simulink model "manual_steer"  (R2022b)
settings: Solver=ode4  StartTime=0.0  StopTime=100  RelTol=1e-3
model workspace (MAT data in the model file):
  x2xx = 0
undefined symbols (not defined in the file or in its folder): axle_rate_limit, BRAKE, brake_lag, brake_rate, DRIVE, KDspd, KIspd, KPspd, Lspd, Nspd, PARSa, PARSu, Q0, QD0, RW, Tb, Tmc, TOTALMASS, Tst, Uspd, v_ref
libraries: CarMaker4SL x72, slpidlib x4, TruckMaker4SL x1, simulink x1
(part 1 of 5)
settings Model: Creator=DJW  LastModifiedBy=14668
settings DebuggingCC: UnconnectedInputMsg=warning  UnconnectedOutputMsg=warning  UnconnectedLineMsg=warning  SFMachineParentedDataDiag=warning
settings ModelReferenceCC: EnableRefExpFcnMdlSchedulingChecks=on

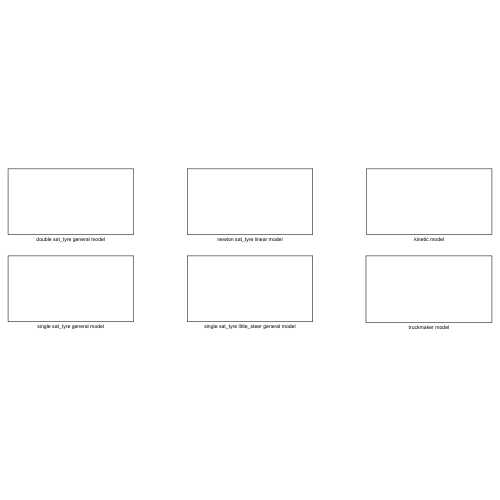
[thumbnail: Simulink's stored preview of the top-level diagram]
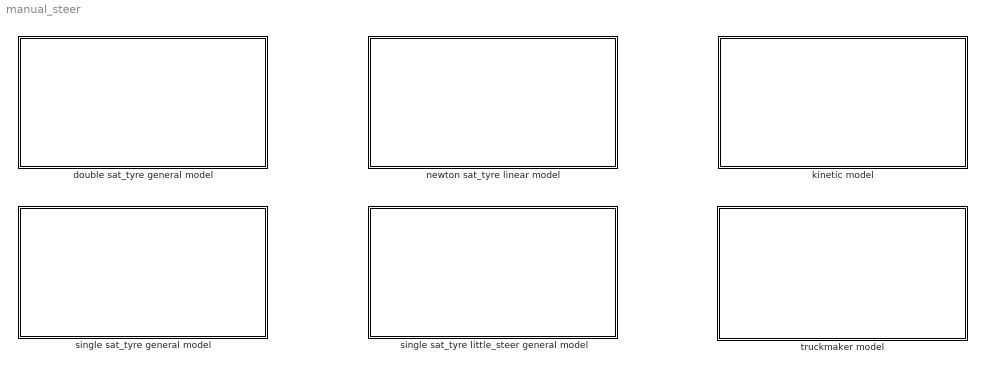
== system manual_steer ==
  double sat_tyre general model : Subsystem
  kinetic model : Subsystem
  newton sat_tyre linear model : Subsystem
  single sat_tyre general model : Subsystem
  single sat_tyre little_steer general model : Subsystem
  truckmaker model : Subsystem

== system manual_steer/double sat_tyre general model ==
  " Motion Controller" : Subsystem  SystemSampleTime=Tmc
  " Motion Controller1" : Subsystem  Commented=on  SystemSampleTime=Tmc
  Clock : Clock
  To Workspace2 : ToWorkspace  VariableName=time  SampleTime=-1
  To Workspace4 : ToWorkspace  VariableName=steer_out  SampleTime=-1
  double-general-lineartyre-nonlinear-constant-matrix : Subsystem  Commented=on
  double-general-lineartyre-variable : Subsystem
  double-general-nonlineartyre-nonlinear-constant-matrix : Subsystem  Commented=on
  double-general-nonlineartyre-nonlinear-variable-matrix : Subsystem  Commented=on
  proc : Subsystem
  single-general-lineartyre-nonlinear-variable-matrix : Subsystem  Commented=on
  wires:
  Clock/1 -> To Workspace2/1
  " Motion Controller"/1(steer6) -> To Workspace4/1, double-general-lineartyre-variable/1(steer)
  " Motion Controller"/2(Fx) -> double-general-lineartyre-variable/2(Fx_in)

== system manual_steer/kinetic model ==
  " Motion Controller No Fx" : Subsystem  SystemSampleTime=Tmc
  Clock : Clock
  To Workspace2 : ToWorkspace  VariableName=time_kinetic  SampleTime=-1
  To Workspace4 : ToWorkspace  VariableName=steer_out_kinetic  SampleTime=-1
  kinetic linear : Subsystem
  proc : Subsystem
  wires:
  Clock/1 -> To Workspace2/1
  " Motion Controller No Fx"/1(steer) -> To Workspace4/1, kinetic linear/1(steer)

== system manual_steer/newton sat_tyre linear model ==
  " Motion Controller No Fx" : Subsystem  SystemSampleTime=Tmc
  Clock : Clock
  To Workspace2 : ToWorkspace  VariableName=time_newton  SampleTime=-1
  To Workspace4 : ToWorkspace  VariableName=steer_out_newton  SampleTime=-1
  newton sat_tyre linear : Subsystem
  proc : Subsystem
  wires:
  Clock/1 -> To Workspace2/1
  " Motion Controller No Fx"/1(steer) -> To Workspace4/1, newton sat_tyre linear/1(steer)

== system manual_steer/single sat_tyre general model ==
  " Motion Controller" : Subsystem  SystemSampleTime=Tmc
  Clock : Clock
  To Workspace2 : ToWorkspace  VariableName=time_single  SampleTime=-1
  To Workspace4 : ToWorkspace  VariableName=steer_out_single  SampleTime=-1
  proc : Subsystem
  single-general-lineartyre-variable : Subsystem
  wires:
  Clock/1 -> To Workspace2/1
  " Motion Controller"/1(steer6) -> To Workspace4/1, single-general-lineartyre-variable/1(steer)
  " Motion Controller"/2(Fx) -> single-general-lineartyre-variable/2(Fx_in)

== system manual_steer/single sat_tyre little_steer general model ==
  " Motion Controller" : Subsystem  SystemSampleTime=Tmc
  Clock : Clock
  To Workspace2 : ToWorkspace  VariableName=time_single_littles  SampleTime=-1
  To Workspace4 : ToWorkspace  VariableName=steer_out_single_littles  SampleTime=-1
  proc : Subsystem
  single-general-lineartyre-little steer-variable : Subsystem
  wires:
  Clock/1 -> To Workspace2/1
  " Motion Controller"/1(steer6) -> To Workspace4/1, single-general-lineartyre-little steer-variable/1(steer)
  " Motion Controller"/2(Fx) -> single-general-lineartyre-little steer-variable/2(Fx_in)

== system manual_steer/truckmaker model ==
  Edit Model Configuration : TruckMaker4SL/Edit Model Configuration  SFunctionModules=''
  Open TruckMaker GUI : Subsystem  LoadFcn=if ~length(which('cmself')), cmenv; end
      settings: OpenFcn=cmblockmagic('gui_fix_display'); TM_Simulink
      mask Display: image(imread('TruckMakerGUI.png'));
  TruckMaker : Subsystem  TreatAsAtomicUnit=on
      mask Display: image(imread('TruckMakerSys.png'));

== system manual_steer/double sat_tyre general model/ Motion Controller ==
  Rate Transition{3..6} (4 alike) : RateTransition
  discrete-time subsystem : Subsystem  TreatAsAtomicUnit=on  SystemSampleTime=Tmc
  steer6 : Outport
  Fx : Outport  Port=2
  wires:
  [q_] -> Rate Transition4/1
  Rate Transition5/1 -> Fx/1
  Rate Transition6/1 -> steer6/1
  [qd_] -> Rate Transition3/1
  discrete-time subsystem/1(steer) -> Rate Transition6/1
  Rate Transition4/1 -> discrete-time subsystem/1(q_in)
  Rate Transition3/1 -> discrete-time subsystem/2(qd_in)
  discrete-time subsystem/2(Fx_input) -> Rate Transition5/1

== system manual_steer/double sat_tyre general model/ Motion Controller1 ==
  Rate Transition6 : RateTransition
  discrete-time subsystem : Subsystem  TreatAsAtomicUnit=on  SystemSampleTime=Tmc
  steer6 : Outport
  wires:
  Rate Transition6/1 -> steer6/1
  discrete-time subsystem/1(steer) -> Rate Transition6/1

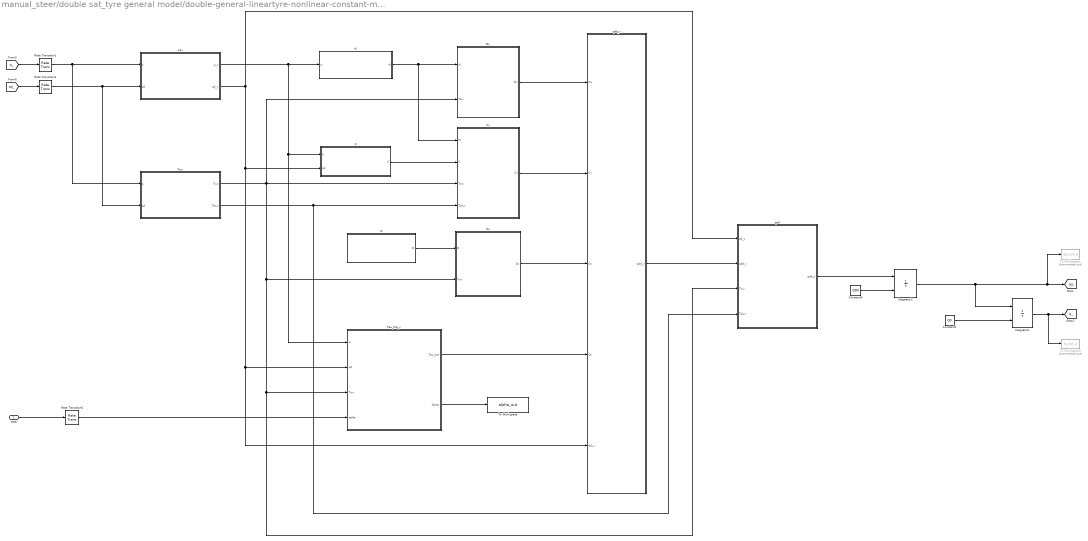
== system manual_steer/double sat_tyre general model/double-general-lineartyre-nonlinear-constant-matrix ==
  steer : Inport
  C : MATLAB Function  TreatAsAtomicUnit=on
  Constant1 : Constant  Value=Q0
  Constant4 : Constant  Value=QD0
  Cv : MATLAB Function  TreatAsAtomicUnit=on
  D : MATLAB Function  TreatAsAtomicUnit=on
  Dv : MATLAB Function  TreatAsAtomicUnit=on
  Integrator1 : Integrator  InitialConditionSource=external  InitialCondition=Q0
  Integrator2 : Integrator  InitialConditionSource=external  InitialCondition=zeros(5,1)
  M : MATLAB Function  TreatAsAtomicUnit=on
  Mv : MATLAB Function  TreatAsAtomicUnit=on
  Rate Transition1 : RateTransition
  Rate Transition2 : RateTransition
  Rate Transition6 : RateTransition
  Tau_tire_v : MATLAB Function  TreatAsAtomicUnit=on
  To Workspace : ToWorkspace  VariableName=alpha_out  SampleTime=-1
  To Workspace1 : ToWorkspace  Commented=on  VariableName=qd_out_4  SampleTime=-1
  To Workspace3 : ToWorkspace  Commented=on  VariableName=q_out_4  SampleTime=-1
  Twv : MATLAB Function  TreatAsAtomicUnit=on
  qdd : MATLAB Function  TreatAsAtomicUnit=on
  qdd_v : MATLAB Function  TreatAsAtomicUnit=on
  w2v : MATLAB Function  TreatAsAtomicUnit=on
  tag scope: q_=global, qd_=global
  wires:
  M/1(M) -> Cv/1(M), Mv/1(M)
  [q_] -> Rate Transition1/1
  [qd_] -> Rate Transition2/1
  Twv/1(Twv) -> qdd/3(Twv), Tau_tire_v/3(Twv), Dv/2(Twv), Cv/3(Twv), Mv/2(Twv)
  C/1(C) -> Cv/2(C)
  Twv/2(Tdwv) -> qdd/4(Tdwv), Cv/4(Tdwv)
  D/1(D) -> Dv/1(D)
  steer/1 -> Rate Transition6/1
  w2v/1(q_v) -> M/1(q), Tau_tire_v/1(q), C/1(q)
  Mv/1(Mv) -> qdd_v/1(Mv)
  Dv/1(Dv) -> qdd_v/3(Dv)
  Cv/1(Cv) -> qdd_v/2(Cv)
  Tau_tire_v/1(Tau_tire) -> qdd_v/4(Qv)
  w2v/2(qd_v) -> qdd/1(qd_v), Tau_tire_v/2(qd), qdd_v/5(qd_v), C/2(qd)
  qdd_v/1(qdd_v) -> qdd/2(qdd_v)
  qdd/1(qdd_n) -> Integrator2/1
  Integrator1/1 -> To Workspace3/1, [q_]
  Integrator2/1 -> To Workspace1/1, [qd_], Integrator1/1
  Tau_tire_v/2(Alpha) -> To Workspace/1
  Constant4/1 -> Integrator2/2
  Constant1/1 -> Integrator1/2
  Rate Transition6/1 -> Tau_tire_v/4(delta)
  Rate Transition1/1 -> Twv/1(q), w2v/1(q)
  Rate Transition2/1 -> Twv/2(qd), w2v/2(qd)

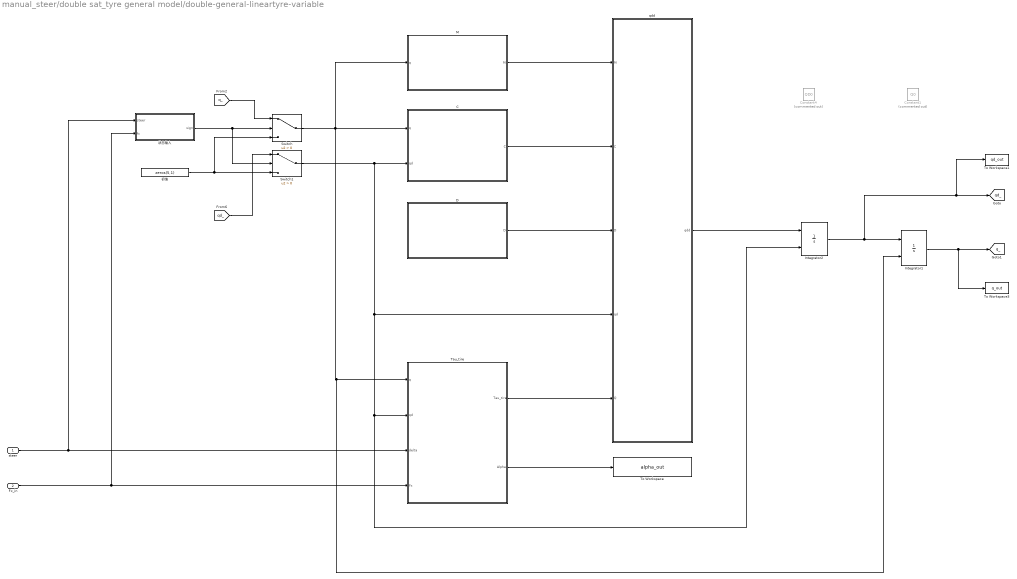
== system manual_steer/double sat_tyre general model/double-general-lineartyre-variable ==
  steer : Inport
  Fx_in : Inport  Port=2
  C : MATLAB Function  TreatAsAtomicUnit=on
  Constant1 : Constant  Commented=on  Value=Q0
  Constant4 : Constant  Commented=on  Value=QD0
  D : MATLAB Function  TreatAsAtomicUnit=on
  Integrator1 : Integrator  InitialConditionSource=external  InitialCondition=Q0
  Integrator2 : Integrator  InitialConditionSource=external  InitialCondition=zeros(5,1)
  M : MATLAB Function  TreatAsAtomicUnit=on
  Switch : Switch  Criteria=u2 > Threshold  SaturateOnIntegerOverflow=off  InputSameDT=off
  Switch1 : Switch  Criteria=u2 > Threshold  SaturateOnIntegerOverflow=off  InputSameDT=off
  Tau_tire : MATLAB Function  TreatAsAtomicUnit=on
  To Workspace : ToWorkspace  VariableName=alpha_out  SampleTime=-1
  To Workspace1 : ToWorkspace  VariableName=qd_out  SampleTime=-1
  To Workspace3 : ToWorkspace  VariableName=q_out  SampleTime=-1
  qdd : MATLAB Function  TreatAsAtomicUnit=on
  初值 : Constant  Value=zeros(5,1)
  状态输入 : MATLAB Function  TreatAsAtomicUnit=on
  tag scope: q_=global, qd_=global
  wires:
  Integrator1/1 -> To Workspace3/1, [q_]
  Fx_in/1 -> 状态输入/2(fx), Tau_tire/4(Fx)
  steer/1 -> 状态输入/1(steer), Tau_tire/3(delta)
  Tau_tire/2(Alpha) -> To Workspace/1
  qdd/1(qdd) -> Integrator2/1
  Integrator2/1 -> To Workspace1/1, [qd_], Integrator1/1
  M/1(M) -> qdd/1(M)
  C/1(C) -> qdd/2(C)
  Tau_tire/1(Tau_tire) -> qdd/5(Q)
  D/1(D) -> qdd/3(D)
  状态输入/1(sign) -> Switch1/2, Switch/2
  初值/1 -> Switch/3, Switch1/3
  Switch/1 -> Integrator1/2, Tau_tire/1(q), M/1(q), C/1(q)
  Switch1/1 -> Integrator2/2, Tau_tire/2(qd), qdd/4(qd), C/2(qd)
  [qd_] -> Switch1/1
  [q_] -> Switch/1

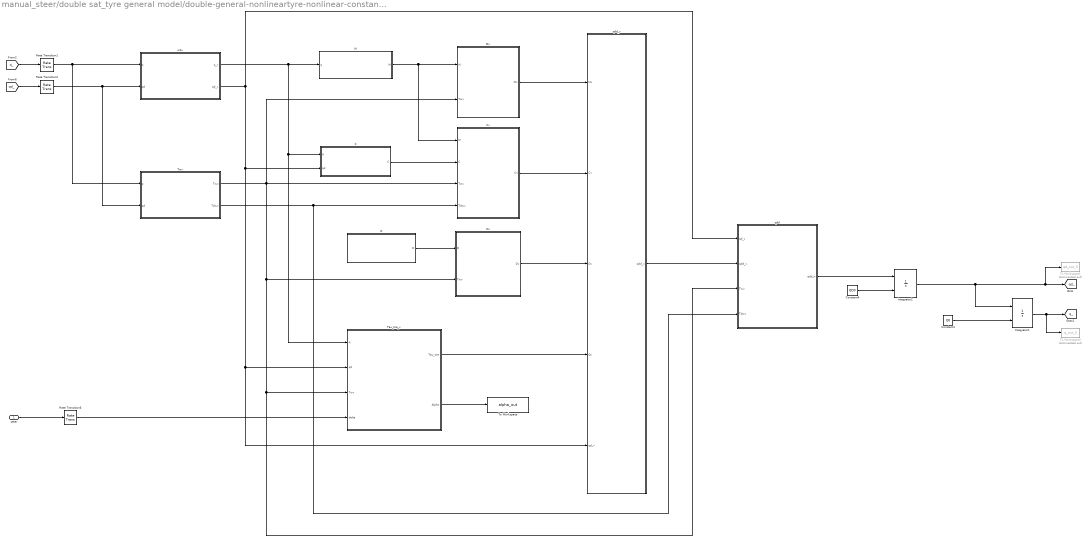
== system manual_steer/double sat_tyre general model/double-general-nonlineartyre-nonlinear-constant-matrix ==
  steer : Inport
  C : MATLAB Function  TreatAsAtomicUnit=on
  Constant1 : Constant  Value=Q0
  Constant4 : Constant  Value=QD0
  Cv : MATLAB Function  TreatAsAtomicUnit=on
  D : MATLAB Function  TreatAsAtomicUnit=on
  Dv : MATLAB Function  TreatAsAtomicUnit=on
  Integrator1 : Integrator  InitialConditionSource=external  InitialCondition=Q0
  Integrator2 : Integrator  InitialConditionSource=external  InitialCondition=zeros(5,1)
  M : MATLAB Function  TreatAsAtomicUnit=on
  Mv : MATLAB Function  TreatAsAtomicUnit=on
  Rate Transition1 : RateTransition
  Rate Transition2 : RateTransition
  Rate Transition6 : RateTransition
  Tau_tire_v : MATLAB Function  TreatAsAtomicUnit=on
  To Workspace : ToWorkspace  VariableName=alpha_out  SampleTime=-1
  To Workspace1 : ToWorkspace  Commented=on  VariableName=qd_out_5  SampleTime=-1
  To Workspace3 : ToWorkspace  Commented=on  VariableName=q_out_5  SampleTime=-1
  Twv : MATLAB Function  TreatAsAtomicUnit=on
  qdd : MATLAB Function  TreatAsAtomicUnit=on
  qdd_v : MATLAB Function  TreatAsAtomicUnit=on
  w2v : MATLAB Function  TreatAsAtomicUnit=on
  tag scope: q_=global, qd_=global
  wires:
  M/1(M) -> Cv/1(M), Mv/1(M)
  [q_] -> Rate Transition1/1
  [qd_] -> Rate Transition2/1
  Twv/1(Twv) -> qdd/3(Twv), Tau_tire_v/3(Twv), Dv/2(Twv), Cv/3(Twv), Mv/2(Twv)
  C/1(C) -> Cv/2(C)
  Twv/2(Tdwv) -> qdd/4(Tdwv), Cv/4(Tdwv)
  D/1(D) -> Dv/1(D)
  steer/1 -> Rate Transition6/1
  w2v/1(q_v) -> M/1(q), Tau_tire_v/1(q), C/1(q)
  Mv/1(Mv) -> qdd_v/1(Mv)
  Dv/1(Dv) -> qdd_v/3(Dv)
  Cv/1(Cv) -> qdd_v/2(Cv)
  Tau_tire_v/1(Tau_tire) -> qdd_v/4(Qv)
  w2v/2(qd_v) -> qdd/1(qd_v), Tau_tire_v/2(qd), qdd_v/5(qd_v), C/2(qd)
  qdd_v/1(qdd_v) -> qdd/2(qdd_v)
  qdd/1(qdd_n) -> Integrator2/1
  Integrator1/1 -> To Workspace3/1, [q_]
  Integrator2/1 -> To Workspace1/1, [qd_], Integrator1/1
  Tau_tire_v/2(Alpha) -> To Workspace/1
  Constant4/1 -> Integrator2/2
  Constant1/1 -> Integrator1/2
  Rate Transition6/1 -> Tau_tire_v/4(delta)
  Rate Transition1/1 -> Twv/1(q), w2v/1(q)
  Rate Transition2/1 -> Twv/2(qd), w2v/2(qd)

== system manual_steer/double sat_tyre general model/double-general-nonlineartyre-nonlinear-variable-matrix ==
  steer : Inport
  Fx_in : Inport  Port=2
  C : MATLAB Function  TreatAsAtomicUnit=on
  Constant1 : Constant  Value=Q0
  Constant4 : Constant  Value=QD0
  D : MATLAB Function  TreatAsAtomicUnit=on
  Integrator1 : Integrator  InitialConditionSource=external  InitialCondition=Q0
  Integrator2 : Integrator  InitialConditionSource=external  InitialCondition=zeros(5,1)
  M : MATLAB Function  TreatAsAtomicUnit=on
  Tau_tire : MATLAB Function  TreatAsAtomicUnit=on
  To Workspace : ToWorkspace  VariableName=alpha_out  SampleTime=-1
  To Workspace1 : ToWorkspace  Commented=on  VariableName=qd_out_6  SampleTime=-1
  To Workspace3 : ToWorkspace  Commented=on  VariableName=q_out_6  SampleTime=-1
  qdd : MATLAB Function  TreatAsAtomicUnit=on
  tag scope: q_=global, qd_=global
  wires:
  Integrator1/1 -> To Workspace3/1, [q_]
  Fx_in/1 -> Tau_tire/4(Fx)
  [q_] -> Tau_tire/1(q), M/1(q), C/1(q)
  [qd_] -> Tau_tire/2(qd), qdd/4(qd), C/2(qd)
  steer/1 -> Tau_tire/3(delta)
  Tau_tire/2(Alpha) -> To Workspace/1
  qdd/1(qdd) -> Integrator2/1
  Integrator2/1 -> To Workspace1/1, [qd_], Integrator1/1
  M/1(M) -> qdd/1(M)
  C/1(C) -> qdd/2(C)
  Tau_tire/1(Tau_tire) -> qdd/5(Q)
  D/1(D) -> qdd/3(D)
  Constant4/1 -> Integrator2/2
  Constant1/1 -> Integrator1/2

== system manual_steer/double sat_tyre general model/proc ==
  Constant1 : Constant  Value=PARSu
  Constant2 : Constant  Value=PARSa
  MatMaker : MATLAB Function  TreatAsAtomicUnit=on
  To Workspace1 : ToWorkspace  VariableName=Va_out  SampleTime=-1
  To Workspace3 : ToWorkspace  VariableName=Vj_out  SampleTime=-1
  To Workspace5 : ToWorkspace  VariableName=Vg_out  SampleTime=-1
  To Workspace6 : ToWorkspace  VariableName=Vgg_out  SampleTime=-1
  To Workspace7 : ToWorkspace  VariableName=Vaa_out  SampleTime=-1
  wires:
  [qd_] -> MatMaker/2(qd)
  MatMaker/1(Va) -> To Workspace1/1
  [q_] -> MatMaker/1(q)
  MatMaker/5(Vgg) -> To Workspace6/1
  MatMaker/3(Vj) -> To Workspace3/1
  Constant1/1 -> MatMaker/3(PARSu)
  MatMaker/4(Vg) -> To Workspace5/1
  Constant2/1 -> MatMaker/4(PARSa)
  MatMaker/2(Vaa) -> To Workspace7/1

== system manual_steer/double sat_tyre general model/single-general-lineartyre-nonlinear-variable-matrix ==
  steer : Inport
  Fx_in : Inport  Port=2
  C : MATLAB Function  TreatAsAtomicUnit=on
  Constant1 : Constant  Value=Q0
  Constant4 : Constant  Value=QD0
  D : MATLAB Function  TreatAsAtomicUnit=on
  Integrator1 : Integrator  InitialConditionSource=external  InitialCondition=Q0
  Integrator2 : Integrator  InitialConditionSource=external  InitialCondition=zeros(5,1)
  M : MATLAB Function  TreatAsAtomicUnit=on
  Tau_tire : MATLAB Function  TreatAsAtomicUnit=on
  To Workspace : ToWorkspace  VariableName=alpha_out  SampleTime=-1
  To Workspace1 : ToWorkspace  Commented=on  VariableName=qd_out_3  SampleTime=-1
  To Workspace3 : ToWorkspace  Commented=on  VariableName=q_out_3  SampleTime=-1
  qdd : MATLAB Function  TreatAsAtomicUnit=on
  tag scope: q_=global, qd_=global
  wires:
  Integrator1/1 -> To Workspace3/1, [q_]
  Fx_in/1 -> Tau_tire/4(Fx)
  [q_] -> Tau_tire/1(q), M/1(q), C/1(q)
  [qd_] -> Tau_tire/2(qd), qdd/4(qd), C/2(qd)
  steer/1 -> Tau_tire/3(delta)
  Tau_tire/2(Alpha) -> To Workspace/1
  qdd/1(qdd) -> Integrator2/1
  M/1(M) -> qdd/1(M)
  C/1(C) -> qdd/2(C)
  Tau_tire/1(Tau_tire) -> qdd/5(Q)
  D/1(D) -> qdd/3(D)
  Constant4/1 -> Integrator2/2
  Constant1/1 -> Integrator1/2
  Integrator2/1 -> To Workspace1/1, [qd_], Integrator1/1

== system manual_steer/kinetic model/ Motion Controller No Fx ==
  note: steering ratio
  Constant3 : Constant  Value=PARSa
  From Workspace : FromWorkspace  VariableName=[tstr_in,str_in]  SampleTime=-1
  From1 : From  Commented=on  GotoTag=qd_kinetic  TagVisibility=global
  From2 : From  Commented=on  GotoTag=q_kinetic  TagVisibility=global
  Gain1 : Gain  Gain=1/20
  MATLAB Function : MATLAB Function  TreatAsAtomicUnit=on
  Rate Limiter1 : RateLimiter  RisingSlewLimit=axle_rate_limit  FallingSlewLimit=-axle_rate_limit  SampleTimeMode=inherited
  Rate Transition1 : RateTransition  Commented=on
  Rate Transition2 : RateTransition
  Rate Transition4 : RateTransition  Commented=on
  steer : Outport
  wires:
  Rate Transition4/1 -> ?
  Rate Limiter1/1 -> Rate Transition2/1
  From2/1 -> Rate Transition4/1
  Constant3/1 -> MATLAB Function/2(PARSa)
  From Workspace/1 -> Gain1/1
  MATLAB Function/1(y) -> Rate Limiter1/1
  From1/1 -> Rate Transition1/1
  Rate Transition2/1 -> steer/1
  Rate Transition1/1 -> ?
  Gain1/1 -> MATLAB Function/1(str1)

== system manual_steer/kinetic model/kinetic linear ==
  steer : Inport
  Constant3 : Constant  Value=[v_ref; 0; 0; 0; 0]
  Constant4 : Constant  Value=v_ref
  Integrator1 : Integrator  InitialConditionSource=external  InitialCondition=Q0
  Switch2 : Switch  Criteria=u2 > Threshold  SaturateOnIntegerOverflow=off  InputSameDT=off
  Switch3 : Switch  Criteria=u2 > Threshold  SaturateOnIntegerOverflow=off  InputSameDT=off
  To Workspace1 : ToWorkspace  VariableName=qd_out_kinetic  SampleTime=-1
  To Workspace3 : ToWorkspace  VariableName=q_out_kinetic  SampleTime=-1
  初值1 : Constant  Value=zeros(5,1)
  状态更新 : MATLAB Function  TreatAsAtomicUnit=on
  状态输入 : MATLAB Function  TreatAsAtomicUnit=on
  tag scope: q_kinetic=global, qd_kinetic=global
  wires:
  Integrator1/1 -> To Workspace3/1, [q_kinetic]
  状态更新/1(qd_output) -> Integrator1/1, To Workspace1/1, [qd_kinetic]
  [qd_kinetic] -> Switch3/1
  [q_kinetic] -> Switch2/1
  状态输入/1(sign) -> Switch3/2, Switch2/2
  初值1/1 -> Switch2/3
  Constant3/1 -> Switch3/3
  steer/1 -> 状态更新/3(delta), 状态输入/1(steer)
  Switch2/1 -> Integrator1/2, 状态更新/1(q)
  Switch3/1 -> 状态更新/4(qd)
  Constant4/1 -> 状态更新/2(v_ref)

== system manual_steer/kinetic model/proc ==
  Constant1 : Constant  Value=PARSu
  Constant2 : Constant  Value=PARSa
  MatMaker : MATLAB Function  TreatAsAtomicUnit=on
  To Workspace1 : ToWorkspace  VariableName=Va_out_kinetic  SampleTime=-1
  To Workspace3 : ToWorkspace  VariableName=Vj_out_kinetic  SampleTime=-1
  To Workspace5 : ToWorkspace  VariableName=Vg_out_kinetic  SampleTime=-1
  To Workspace6 : ToWorkspace  VariableName=Vgg_out_kinetic  SampleTime=-1
  To Workspace7 : ToWorkspace  VariableName=Vaa_out_kinetic  SampleTime=-1
  wires:
  [qd_kinetic] -> MatMaker/2(qd)
  MatMaker/1(Va) -> To Workspace1/1
  [q_kinetic] -> MatMaker/1(q)
  MatMaker/5(Vgg) -> To Workspace6/1
  MatMaker/3(Vj) -> To Workspace3/1
  Constant1/1 -> MatMaker/3(PARSu)
  MatMaker/4(Vg) -> To Workspace5/1
  Constant2/1 -> MatMaker/4(PARSa)
  MatMaker/2(Vaa) -> To Workspace7/1

== system manual_steer/newton sat_tyre linear model/ Motion Controller No Fx ==
  note: steering ratio
  Constant3 : Constant  Value=PARSa
  Digital Clock1 : DigitalClock  Commented=on  SampleTime=-1
  From Workspace : FromWorkspace  VariableName=[tstr_in,str_in]  SampleTime=-1
  Gain1 : Gain  Gain=1/20
  MATLAB Function : MATLAB Function  TreatAsAtomicUnit=on
  Rate Limiter1 : RateLimiter  RisingSlewLimit=axle_rate_limit  FallingSlewLimit=-axle_rate_limit  SampleTimeMode=inherited
  Rate Transition1 : RateTransition
  Rate Transition2 : RateTransition
  Rate Transition4 : RateTransition
  To Workspace3 : ToWorkspace  Commented=on  VariableName=tdig_out_newton  SampleTime=-1
  steer : Outport
  wires:
  MATLAB Function/1(y) -> Rate Limiter1/1
  Gain1/1 -> MATLAB Function/1(str1)
  Constant3/1 -> MATLAB Function/2(PARSa)
  From Workspace/1 -> Gain1/1
  Digital Clock1/1 -> To Workspace3/1
  Rate Limiter1/1 -> Rate Transition2/1
  Rate Transition4/1 -> MATLAB Function/3(q)
  [q_newton] -> Rate Transition4/1
  Rate Transition2/1 -> steer/1
  Rate Transition1/1 -> MATLAB Function/4(qd)
  [qd_newton] -> Rate Transition1/1

== system manual_steer/newton sat_tyre linear model/newton sat_tyre linear ==
  steer : Inport
  Constant2 : Constant  Value=[v_ref; 0; 0; 0; 0]
  Integrator1 : Integrator  InitialConditionSource=external  InitialCondition=Q0
  Integrator2 : Integrator  InitialConditionSource=external  InitialCondition=zeros(5,1)
  Switch : Switch  Criteria=u2 > Threshold  SaturateOnIntegerOverflow=off  InputSameDT=off
  Switch1 : Switch  Criteria=u2 > Threshold  SaturateOnIntegerOverflow=off  InputSameDT=off
  To Workspace1 : ToWorkspace  VariableName=qd_out_newton  SampleTime=-1
  To Workspace3 : ToWorkspace  VariableName=q_out_newton  SampleTime=-1
  To Workspace5 : ToWorkspace  VariableName=qdd_out_newton  SampleTime=-1
      settings: Save2DSignal=2-D array (concatenate along first dimension)
  get state : MATLAB Function  TreatAsAtomicUnit=on
  get tyre f : MATLAB Function  TreatAsAtomicUnit=on
  state_update : MATLAB Function  TreatAsAtomicUnit=on
  初值 : Constant  Value=zeros(5,1)
  状态输入 : MATLAB Function  TreatAsAtomicUnit=on
  tag scope: q_newton=global, qd_newton=global
  wires:
  Integrator1/1 -> To Workspace3/1, [q_newton]
  steer/1 -> get tyre f/3(delta_input), 状态输入/1(steer)
  Integrator2/1 -> To Workspace1/1, [qd_newton], Integrator1/1
  状态输入/1(sign) -> Switch1/2, Switch/2
  初值/1 -> Switch/3
  [qd_newton] -> Switch1/1
  [q_newton] -> Switch/1
  Constant2/1 -> Switch1/3
  Switch/1 -> get state/1(q_input), state_update/2(q_input), get tyre f/1(q_input), Integrator1/2
  Switch1/1 -> get state/2(qd_input), state_update/3(qd_input), Integrator2/2, get tyre f/2(qd_input)
  get tyre f/1(yij) -> state_update/4(yij)
  get state/1(x) -> state_update/1(x)
  state_update/1(qdd_output) -> To Workspace5/1, Integrator2/1

== system manual_steer/newton sat_tyre linear model/proc ==
  Constant1 : Constant  Value=PARSu
  Constant2 : Constant  Value=PARSa
  MatMaker : MATLAB Function  TreatAsAtomicUnit=on
  To Workspace1 : ToWorkspace  VariableName=Va_out_newton  SampleTime=-1
  To Workspace3 : ToWorkspace  VariableName=Vj_out_newton  SampleTime=-1
  To Workspace5 : ToWorkspace  VariableName=Vg_out_newton  SampleTime=-1
  To Workspace6 : ToWorkspace  VariableName=Vgg_out_newton  SampleTime=-1
  To Workspace7 : ToWorkspace  VariableName=Vaa_out_newton  SampleTime=-1
  wires:
  [qd_newton] -> MatMaker/2(qd)
  MatMaker/1(Va) -> To Workspace1/1
  [q_newton] -> MatMaker/1(q)
  MatMaker/5(Vgg) -> To Workspace6/1
  MatMaker/3(Vj) -> To Workspace3/1
  Constant1/1 -> MatMaker/3(PARSu)
  MatMaker/4(Vg) -> To Workspace5/1
  Constant2/1 -> MatMaker/4(PARSa)
  MatMaker/2(Vaa) -> To Workspace7/1

== system manual_steer/single sat_tyre general model/ Motion Controller ==
  Rate Transition{3..6} (4 alike) : RateTransition
  discrete-time subsystem single : Subsystem  TreatAsAtomicUnit=on  SystemSampleTime=Tmc
  steer6 : Outport
  Fx : Outport  Port=2
  wires:
  [q_single] -> Rate Transition4/1
  Rate Transition5/1 -> Fx/1
  Rate Transition6/1 -> steer6/1
  [qd_single] -> Rate Transition3/1
  discrete-time subsystem single/1(steer) -> Rate Transition6/1
  Rate Transition4/1 -> discrete-time subsystem single/1(q_in)
  Rate Transition3/1 -> discrete-time subsystem single/2(qd_in)
  discrete-time subsystem single/2(Fx_input) -> Rate Transition5/1

== system manual_steer/single sat_tyre general model/proc ==
  Constant1 : Constant  Value=PARSu
  Constant2 : Constant  Value=PARSa
  MatMaker : MATLAB Function  TreatAsAtomicUnit=on
  To Workspace1 : ToWorkspace  VariableName=Va_out_single  SampleTime=-1
  To Workspace3 : ToWorkspace  VariableName=Vj_out_single  SampleTime=-1
  To Workspace5 : ToWorkspace  VariableName=Vg_out_single  SampleTime=-1
  To Workspace6 : ToWorkspace  VariableName=Vgg_out_single  SampleTime=-1
  To Workspace7 : ToWorkspace  VariableName=Vaa_out_single  SampleTime=-1
  wires:
  [qd_single] -> MatMaker/2(qd)
  MatMaker/1(Va) -> To Workspace1/1
  [q_single] -> MatMaker/1(q)
  MatMaker/5(Vgg) -> To Workspace6/1
  MatMaker/3(Vj) -> To Workspace3/1
  Constant1/1 -> MatMaker/3(PARSu)
  MatMaker/4(Vg) -> To Workspace5/1
  Constant2/1 -> MatMaker/4(PARSa)
  MatMaker/2(Vaa) -> To Workspace7/1

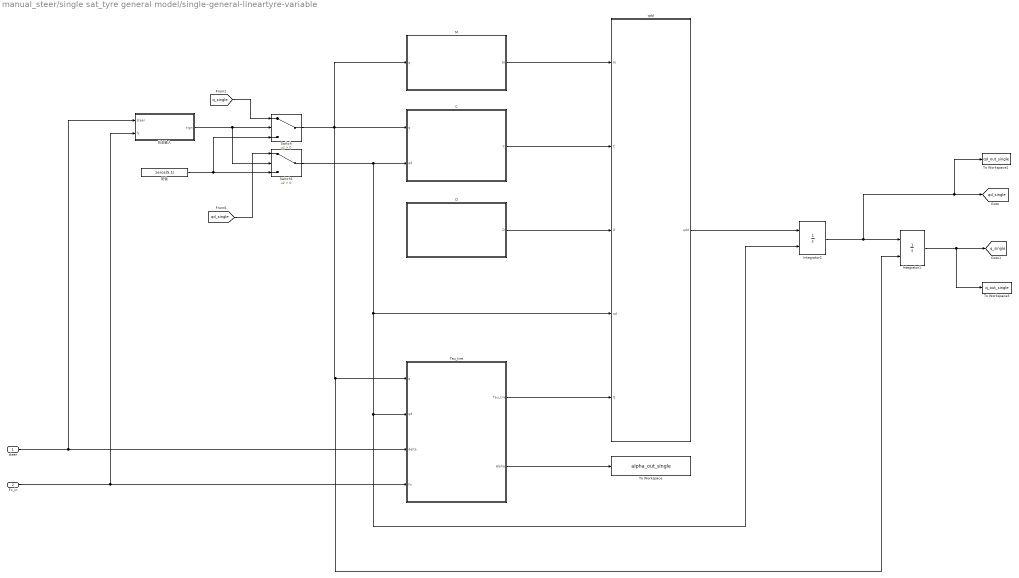
== system manual_steer/single sat_tyre general model/single-general-lineartyre-variable ==
  steer : Inport
  Fx_in : Inport  Port=2
  C : MATLAB Function  TreatAsAtomicUnit=on
  D : MATLAB Function  TreatAsAtomicUnit=on
  Integrator1 : Integrator  InitialConditionSource=external  InitialCondition=Q0
  Integrator2 : Integrator  InitialConditionSource=external  InitialCondition=zeros(5,1)
  M : MATLAB Function  TreatAsAtomicUnit=on
  Switch : Switch  Criteria=u2 > Threshold  SaturateOnIntegerOverflow=off  InputSameDT=off
  Switch1 : Switch  Criteria=u2 > Threshold  SaturateOnIntegerOverflow=off  InputSameDT=off
  Tau_tire : MATLAB Function  TreatAsAtomicUnit=on
  To Workspace : ToWorkspace  VariableName=alpha_out_single  SampleTime=-1
  To Workspace1 : ToWorkspace  VariableName=qd_out_single  SampleTime=-1
  To Workspace3 : ToWorkspace  VariableName=q_out_single  SampleTime=-1
  qdd : MATLAB Function  TreatAsAtomicUnit=on
  初值 : Constant  Value=zeros(5,1)
  状态输入 : MATLAB Function  TreatAsAtomicUnit=on
  tag scope: q_single=global, qd_single=global
  wires:
  Integrator1/1 -> To Workspace3/1, [q_single]
  Fx_in/1 -> 状态输入/2(fx), Tau_tire/4(Fx)
  steer/1 -> 状态输入/1(steer), Tau_tire/3(delta)
  Tau_tire/2(Alpha) -> To Workspace/1
  qdd/1(qdd) -> Integrator2/1
  Integrator2/1 -> To Workspace1/1, [qd_single], Integrator1/1
  M/1(M) -> qdd/1(M)
  C/1(C) -> qdd/2(C)
  Tau_tire/1(Tau_tire) -> qdd/5(Q)
  D/1(D) -> qdd/3(D)
  状态输入/1(sign) -> Switch1/2, Switch/2
  初值/1 -> Switch/3, Switch1/3
  Switch/1 -> Integrator1/2, Tau_tire/1(q), M/1(q), C/1(q)
  Switch1/1 -> Integrator2/2, Tau_tire/2(qd), qdd/4(qd), C/2(qd)
  [qd_single] -> Switch1/1
  [q_single] -> Switch/1

== system manual_steer/single sat_tyre little_steer general model/ Motion Controller ==
  Rate Transition{3..6} (4 alike) : RateTransition
  discrete-time subsystem single little steer : Subsystem  TreatAsAtomicUnit=on  SystemSampleTime=Tmc
  steer6 : Outport
  Fx : Outport  Port=2
  wires:
  [q_single_littles] -> Rate Transition4/1
  Rate Transition5/1 -> Fx/1
  Rate Transition6/1 -> steer6/1
  [qd_single_littles] -> Rate Transition3/1
  discrete-time subsystem single little steer/1(steer) -> Rate Transition6/1
  Rate Transition4/1 -> discrete-time subsystem single little steer/1(q_in)
  Rate Transition3/1 -> discrete-time subsystem single little steer/2(qd_in)
  discrete-time subsystem single little steer/2(Fx_input) -> Rate Transition5/1

== system manual_steer/single sat_tyre little_steer general model/proc ==
  Constant1 : Constant  Value=PARSu
  Constant2 : Constant  Value=PARSa
  MatMaker : MATLAB Function  TreatAsAtomicUnit=on
  To Workspace1 : ToWorkspace  VariableName=Va_out_single_littles  SampleTime=-1
  To Workspace3 : ToWorkspace  VariableName=Vj_out_single_littles  SampleTime=-1
  To Workspace5 : ToWorkspace  VariableName=Vg_out_single_littles  SampleTime=-1
  To Workspace6 : ToWorkspace  VariableName=Vgg_out_single_littles  SampleTime=-1
  To Workspace7 : ToWorkspace  VariableName=Vaa_out_single_littles  SampleTime=-1
  wires:
  [qd_single_littles] -> MatMaker/2(qd)
  MatMaker/1(Va) -> To Workspace1/1
  [q_single_littles] -> MatMaker/1(q)
  MatMaker/5(Vgg) -> To Workspace6/1
  MatMaker/3(Vj) -> To Workspace3/1
  Constant1/1 -> MatMaker/3(PARSu)
  MatMaker/4(Vg) -> To Workspace5/1
  Constant2/1 -> MatMaker/4(PARSa)
  MatMaker/2(Vaa) -> To Workspace7/1

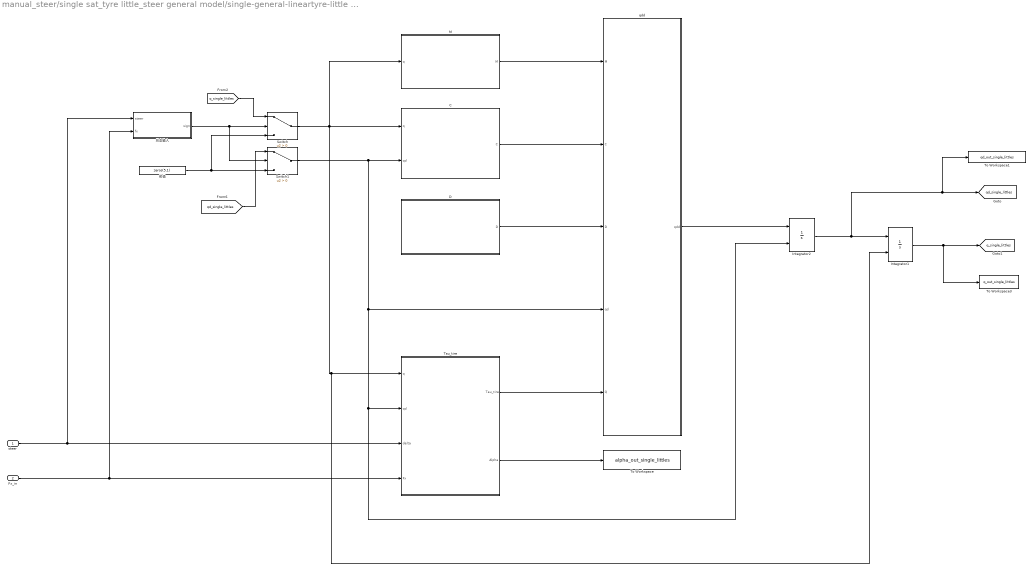
== system manual_steer/single sat_tyre little_steer general model/single-general-lineartyre-little steer-variable ==
  steer : Inport
  Fx_in : Inport  Port=2
  C : MATLAB Function  TreatAsAtomicUnit=on
  D : MATLAB Function  TreatAsAtomicUnit=on
  Integrator1 : Integrator  InitialConditionSource=external  InitialCondition=Q0
  Integrator2 : Integrator  InitialConditionSource=external  InitialCondition=zeros(5,1)
  M : MATLAB Function  TreatAsAtomicUnit=on
  Switch : Switch  Criteria=u2 > Threshold  SaturateOnIntegerOverflow=off  InputSameDT=off
  Switch1 : Switch  Criteria=u2 > Threshold  SaturateOnIntegerOverflow=off  InputSameDT=off
  Tau_tire : MATLAB Function  TreatAsAtomicUnit=on
  To Workspace : ToWorkspace  VariableName=alpha_out_single_littles  SampleTime=-1
  To Workspace1 : ToWorkspace  VariableName=qd_out_single_littles  SampleTime=-1
  To Workspace3 : ToWorkspace  VariableName=q_out_single_littles  SampleTime=-1
  qdd : MATLAB Function  TreatAsAtomicUnit=on
  初值 : Constant  Value=zeros(5,1)
  状态输入 : MATLAB Function  TreatAsAtomicUnit=on
  tag scope: q_single_littles=global, qd_single_littles=global
  wires:
  Integrator1/1 -> To Workspace3/1, [q_single_littles]
  Fx_in/1 -> 状态输入/2(fx), Tau_tire/4(Fx)
  steer/1 -> 状态输入/1(steer), Tau_tire/3(delta)
  Tau_tire/2(Alpha) -> To Workspace/1
  qdd/1(qdd) -> Integrator2/1
  Integrator2/1 -> To Workspace1/1, [qd_single_littles], Integrator1/1
  M/1(M) -> qdd/1(M)
  C/1(C) -> qdd/2(C)
  Tau_tire/1(Tau_tire) -> qdd/5(Q)
  D/1(D) -> qdd/3(D)
  状态输入/1(sign) -> Switch1/2, Switch/2
  初值/1 -> Switch/3, Switch1/3
  Switch/1 -> Integrator1/2, Tau_tire/1(q), M/1(q), C/1(q)
  Switch1/1 -> Integrator2/2, Tau_tire/2(qd), qdd/4(qd), C/2(qd)
  [qd_single_littles] -> Switch1/1
  [q_single_littles] -> Switch/1

== system manual_steer/truckmaker model/Open TruckMaker GUI ==
  S-Function : S-Function  FunctionName=cm_gui  SFunctionDeploymentMode=off  EnableBusSupport=off

== system manual_steer/truckmaker model/TruckMaker ==
  note: main code in IPG Vehicle
  CM_FIRST : Subsystem
  CM_LAST : Subsystem
  DrivMan : Subsystem
  Ground : Ground
  IPG Vehicle : Subsystem  TreatAsAtomicUnit=on
  Terminator : Terminator
  VehicleControl : Subsystem
  wires:
  VehicleControl/2(Vhcl.Model.Source) -> IPG Vehicle/2(Vhcl.Model.Source)
  VehicleControl/7(VhclCtrl.PT) -> IPG Vehicle/7(VhclCtrl.PT)
  VehicleControl/6(VhclCtrl.Brake) -> IPG Vehicle/6(VhclCtrl.Brake)
  VehicleControl/5(Vhcl.Misc) -> IPG Vehicle/5(Vhcl.Misc)
  VehicleControl/4(Vhcl.Wheel.In) -> IPG Vehicle/4(Vhcl.Wheel.In)
  VehicleControl/3(VhclCtrl.Steering) -> IPG Vehicle/3(VhclCtrl.Steering)
  VehicleControl/1(Sync_Out) -> IPG Vehicle/1(Sync_In)
  IPG Vehicle/1(Sync_Out) -> CM_LAST/1(Sync_In)
  Ground/1 -> CM_FIRST/1(Sync_In)
  CM_LAST/1(Sync_Out) -> Terminator/1
  CM_FIRST/1(Sync_Out) -> DrivMan/1(Sync_In)
  CM_FIRST/2(Env.Misc) -> DrivMan/2(Env.Misc)
  DrivMan/1(Sync_Out) -> VehicleControl/1(Sync_In)
  DrivMan/2(DrivMan.Out) -> VehicleControl/2(DrivMan.In)

== system manual_steer/double sat_tyre general model/ Motion Controller/discrete-time subsystem ==
  note: steering ratio
  note: OL steering wheel angle in rad
  q_in : Inport
  qd_in : Inport  Port=2
  " PARSu" : Constant  Value=PARSu
  Constant2 : Constant  Value=v_ref
  Constant3 : Constant  Value=PARSa
  Digital Clock1 : DigitalClock  Commented=on  SampleTime=-1
  From Workspace : FromWorkspace  VariableName=[tstr_in,str_in]  SampleTime=-1
  Gain1 : Gain  Gain=1/20
  MATLAB Function : MATLAB Function  TreatAsAtomicUnit=on
  MATLAB Function1 : MATLAB Function  TreatAsAtomicUnit=on
  PARSa : Constant  Value=PARSa
  PID Controller : slpidlib/PID Controller  Controller=PID  Form=Parallel  TimeDomain=Discrete-time  UseExternalTs=off  SampleTime=-1  IntegratorMethod=Forward Euler  FilterMethod=Forward Euler  ControllerParametersSource=internal  P=KPspd  I=KIspd  UseKiTs=off  D=KDspd  N=Nspd  UseFilter=on  TunerSelectOption=Transfer Function Based (PID Tuner App)  InitialConditionSource=internal  InitialConditionForIntegrator=0  InitialConditionForFilter=0  DifferentiatorICPrevScaledInput=0  ExternalReset=none  TrackingMode=off  Kt=1  LimitOutput=on  SatLimitsSource=internal  UpperSaturationLimit=Uspd  LowerSaturationLimit=Lspd  LinearizeAsGain=on  AntiWindupMode=clamping  Kb=1  LimitIntegrator=off  UpperIntegratorSaturationLimit=inf  LowerIntegratorSaturationLimit=-inf  POutMin=[]  POutMax=[]  IOutMin=[]  IOutMax=[]  DOutMin=[]  DOutMax=[]  NOutMin=[]  NOutMax=[]  SumOutMin=[]  SumOutMax=[]  SaturationOutMin=[]  SaturationOutMax=[]  PParamMin=[]  PParamMax=[]  IParamMin=[]  IParamMax=[]  DParamMin=[]  DParamMax=[]  NParamMin=[]  NParamMax=[]  KbParamMin=[]  KbParamMax=[]  KtParamMin=[]  KtParamMax=[]  KbOutMin=[]  KbOutMax=[]  KtOutMin=[]  KtOutMax=[]  IntegratorOutMin=[]  IntegratorOutMax=[]  FilterOutMin=[]  FilterOutMax=[]  SumI1OutMin=[]  SumI1OutMax=[]  SumI2OutMin=[]  SumI2OutMax=[]  SumI3OutMin=[]  SumI3OutMax=[]  SumI4OutMin=[]  SumI4OutMax=[]  SumDOutMin=[]  SumDOutMax=[]  DifferentiatorOutMin=[]  DifferentiatorOutMax=[]  FilterDiffOutCoefMin=[]  FilterDiffOutCoefMax=[]  ReciprocalOutMin=[]  ReciprocalOutMax=[]  SumDenOutMin=[]  SumDenOutMax=[]  SumNumOutMin=[]  SumNumOutMax=[]  DivideOutMin=[]  DivideOutMax=[]  UdiffTsProdOutMin=[]  UdiffTsProdOutMax=[]  NTsProdOutMin=[]  NTsProdOutMax=[]  UintegralTsProdOutMin=[]  UintegralTsProdOutMax=[]  UngainTsProdOutMin=[]  UngainTsProdOutMax=[]  ClampingZeroOutDataTypeStr=Inherit: Inherit via back propagation  ClampingZeroOutMin=[]  ClampingZeroOutMax=[]  FilterDenConstantOutDataTypeStr=Inherit: Inherit via back propagation  FilterDenConstantOutMin=[]  FilterDenConstantOutMax=[]  PCopyOutDataTypeStr=Inherit: Inherit via back propagation  PCopyOutMin=[]  PCopyOutMax=[]  NCopyOutDataTypeStr=Inherit: Inherit via back propagation  NCopyOutMin=[]  NCopyOutMax=[]  IntegratorContinuousStateAttributes=''  IntegratorStateMustResolveToSignalObject=off  IntegratorRTWStateStorageClass=Auto  FilterContinuousStateAttributes=''  FilterStateMustResolveToSignalObject=off  FilterRTWStateStorageClass=Auto  ParallelPVariant=InternalParameters  IdealPVariant=Disabled  IVariant=InternalParameters  DVariant=InternalParameters  IntegratorVariant=Discrete  SatVariant=Enabled  AWVariant=DiscClampingParallel  PCopyVariant=Disabled  TRVariant=Disabled  FdbkBlocksVariant=Forward  IdealPFdbkVariant=Disabled  SatFdbkVariant=Disabled  DerivativeFilterVariant=ForwardEulerFilter  NVariant=InternalParameters  NCopyVariant=Disabled  FilterICVariant=InternalICsFilter  IntegratorICVariant=InternalICs  ExternalResetVariant=Disabled  TRSumVariant=Passthrough  SumFdbkVariant=Disabled  SumVariant=Sum_PID  TsampFilterVariant=InternalTs  TsampNgainVariant=Passthrough  TsampIntegralVariant=Passthrough  ExternalSaturationOutDataTypeStr=Inherit: Same as second input
  Rate Limiter1 : RateLimiter  RisingSlewLimit=axle_rate_limit  FallingSlewLimit=-axle_rate_limit  SampleTimeMode=inherited
  Scope : Scope
  Sum : Sum  Inputs=|-+
  To Workspace2 : ToWorkspace  VariableName=U_out  SampleTime=-1
  To Workspace3 : ToWorkspace  Commented=on  VariableName=tdig_out1  SampleTime=-1
  getU : MATLAB Function  TreatAsAtomicUnit=on
  steer : Outport
  Fx_input : Outport  Port=2  VectorParamsAs1DForOutWhenUnconnected=off
  wires:
  q_in/1 -> getU/1(q)
  qd_in/1 -> getU/2(qd)
  getU/1(U) -> To Workspace2/1, Sum/1
  Digital Clock1/1 -> To Workspace3/1
  From Workspace/1 -> Gain1/1
  Gain1/1 -> Scope/1, MATLAB Function/1(str1)
  MATLAB Function/1(y) -> Rate Limiter1/1
  Constant3/1 -> MATLAB Function/2(PARSa)
  Rate Limiter1/1 -> steer/1
  MATLAB Function1/1(y) -> Fx_input/1
  " PARSu"/1 -> MATLAB Function1/2(PARSu)
  PARSa/1 -> MATLAB Function1/3(PARSa)
  Sum/1 -> PID Controller/1
  PID Controller/1 -> MATLAB Function1/1(adem)
  Constant2/1 -> Sum/2

== system manual_steer/double sat_tyre general model/ Motion Controller1/discrete-time subsystem ==
  note: steering ratio
  note: OL steering wheel angle in rad
  Constant3 : Constant  Value=PARSa
  Digital Clock1 : DigitalClock  SampleTime=-1
  From Workspace : FromWorkspace  VariableName=[tstr_in,str_in]  SampleTime=-1
  Gain1 : Gain  Gain=1/20
  MATLAB Function : MATLAB Function  TreatAsAtomicUnit=on
  Rate Limiter1 : RateLimiter  RisingSlewLimit=axle_rate_limit  FallingSlewLimit=-axle_rate_limit  SampleTimeMode=inherited
  To Workspace3 : ToWorkspace  VariableName=tdig_out1  SampleTime=-1
  steer : Outport
  wires:
  Digital Clock1/1 -> To Workspace3/1
  From Workspace/1 -> Gain1/1
  Gain1/1 -> MATLAB Function/1(str1)
  MATLAB Function/1(y) -> Rate Limiter1/1
  Constant3/1 -> MATLAB Function/2(PARSa)
  Rate Limiter1/1 -> steer/1

== system manual_steer/single sat_tyre general model/ Motion Controller/discrete-time subsystem single ==
  note: steering ratio
  note: OL steering wheel angle in rad
  q_in : Inport
  qd_in : Inport  Port=2
  " PARSu" : Constant  Value=PARSu
  Constant2 : Constant  Value=v_ref
  Constant3 : Constant  Value=PARSa
  Digital Clock1 : DigitalClock  Commented=on  SampleTime=-1
  From Workspace : FromWorkspace  VariableName=[tstr_in,str_in]  SampleTime=-1
  Gain1 : Gain  Gain=1/20
  MATLAB Function : MATLAB Function  TreatAsAtomicUnit=on
  MATLAB Function1 : MATLAB Function  TreatAsAtomicUnit=on
  PARSa : Constant  Value=PARSa
  PID Controller : slpidlib/PID Controller  Controller=PID  Form=Parallel  TimeDomain=Discrete-time  UseExternalTs=off  SampleTime=-1  IntegratorMethod=Forward Euler  FilterMethod=Forward Euler  ControllerParametersSource=internal  P=KPspd  I=KIspd  UseKiTs=off  D=KDspd  N=Nspd  UseFilter=on  TunerSelectOption=Transfer Function Based (PID Tuner App)  InitialConditionSource=internal  InitialConditionForIntegrator=0  InitialConditionForFilter=0  DifferentiatorICPrevScaledInput=0  ExternalReset=none  TrackingMode=off  Kt=1  LimitOutput=on  SatLimitsSource=internal  UpperSaturationLimit=Uspd  LowerSaturationLimit=Lspd  LinearizeAsGain=on  AntiWindupMode=clamping  Kb=1  LimitIntegrator=off  UpperIntegratorSaturationLimit=inf  LowerIntegratorSaturationLimit=-inf  POutMin=[]  POutMax=[]  IOutMin=[]  IOutMax=[]  DOutMin=[]  DOutMax=[]  NOutMin=[]  NOutMax=[]  SumOutMin=[]  SumOutMax=[]  SaturationOutMin=[]  SaturationOutMax=[]  PParamMin=[]  PParamMax=[]  IParamMin=[]  IParamMax=[]  DParamMin=[]  DParamMax=[]  NParamMin=[]  NParamMax=[]  KbParamMin=[]  KbParamMax=[]  KtParamMin=[]  KtParamMax=[]  KbOutMin=[]  KbOutMax=[]  KtOutMin=[]  KtOutMax=[]  IntegratorOutMin=[]  IntegratorOutMax=[]  FilterOutMin=[]  FilterOutMax=[]  SumI1OutMin=[]  SumI1OutMax=[]  SumI2OutMin=[]  SumI2OutMax=[]  SumI3OutMin=[]  SumI3OutMax=[]  SumI4OutMin=[]  SumI4OutMax=[]  SumDOutMin=[]  SumDOutMax=[]  DifferentiatorOutMin=[]  DifferentiatorOutMax=[]  FilterDiffOutCoefMin=[]  FilterDiffOutCoefMax=[]  ReciprocalOutMin=[]  ReciprocalOutMax=[]  SumDenOutMin=[]  SumDenOutMax=[]  SumNumOutMin=[]  SumNumOutMax=[]  DivideOutMin=[]  DivideOutMax=[]  UdiffTsProdOutMin=[]  UdiffTsProdOutMax=[]  NTsProdOutMin=[]  NTsProdOutMax=[]  UintegralTsProdOutMin=[]  UintegralTsProdOutMax=[]  UngainTsProdOutMin=[]  UngainTsProdOutMax=[]  ClampingZeroOutDataTypeStr=Inherit: Inherit via back propagation  ClampingZeroOutMin=[]  ClampingZeroOutMax=[]  FilterDenConstantOutDataTypeStr=Inherit: Inherit via back propagation  FilterDenConstantOutMin=[]  FilterDenConstantOutMax=[]  PCopyOutDataTypeStr=Inherit: Inherit via back propagation  PCopyOutMin=[]  PCopyOutMax=[]  NCopyOutDataTypeStr=Inherit: Inherit via back propagation  NCopyOutMin=[]  NCopyOutMax=[]  IntegratorContinuousStateAttributes=''  IntegratorStateMustResolveToSignalObject=off  IntegratorRTWStateStorageClass=Auto  FilterContinuousStateAttributes=''  FilterStateMustResolveToSignalObject=off  FilterRTWStateStorageClass=Auto  ParallelPVariant=InternalParameters  IdealPVariant=Disabled  IVariant=InternalParameters  DVariant=InternalParameters  IntegratorVariant=Discrete  SatVariant=Enabled  AWVariant=DiscClampingParallel  PCopyVariant=Disabled  TRVariant=Disabled  FdbkBlocksVariant=Forward  IdealPFdbkVariant=Disabled  SatFdbkVariant=Disabled  DerivativeFilterVariant=ForwardEulerFilter  NVariant=InternalParameters  NCopyVariant=Disabled  FilterICVariant=InternalICsFilter  IntegratorICVariant=InternalICs  ExternalResetVariant=Disabled  TRSumVariant=Passthrough  SumFdbkVariant=Disabled  SumVariant=Sum_PID  TsampFilterVariant=InternalTs  TsampNgainVariant=Passthrough  TsampIntegralVariant=Passthrough  ExternalSaturationOutDataTypeStr=Inherit: Same as second input
  Rate Limiter1 : RateLimiter  RisingSlewLimit=axle_rate_limit  FallingSlewLimit=-axle_rate_limit  SampleTimeMode=inherited
  Scope : Scope
  Sum : Sum  Inputs=|-+
  To Workspace2 : ToWorkspace  VariableName=U_out_single  SampleTime=-1
  To Workspace3 : ToWorkspace  Commented=on  VariableName=tdig_out_single  SampleTime=-1
  getU : MATLAB Function  TreatAsAtomicUnit=on
  steer : Outport
  Fx_input : Outport  Port=2  VectorParamsAs1DForOutWhenUnconnected=off
  wires:
  q_in/1 -> getU/1(q)
  qd_in/1 -> getU/2(qd)
  getU/1(U) -> To Workspace2/1, Sum/1
  Digital Clock1/1 -> To Workspace3/1
  From Workspace/1 -> Gain1/1
  Gain1/1 -> Scope/1, MATLAB Function/1(str1)
  MATLAB Function/1(y) -> Rate Limiter1/1
  Constant3/1 -> MATLAB Function/2(PARSa)
  Rate Limiter1/1 -> steer/1
  MATLAB Function1/1(y) -> Fx_input/1
  " PARSu"/1 -> MATLAB Function1/2(PARSu)
  PARSa/1 -> MATLAB Function1/3(PARSa)
  Sum/1 -> PID Controller/1
  PID Controller/1 -> MATLAB Function1/1(adem)
  Constant2/1 -> Sum/2

== system manual_steer/single sat_tyre little_steer general model/ Motion Controller/discrete-time subsystem single little steer ==
  note: steering ratio
  note: OL steering wheel angle in rad
  q_in : Inport
  qd_in : Inport  Port=2
  " PARSu" : Constant  Value=PARSu
  Constant2 : Constant  Value=v_ref
  Constant3 : Constant  Value=PARSa
  Digital Clock1 : DigitalClock  Commented=on  SampleTime=-1
  From Workspace : FromWorkspace  VariableName=[tstr_in,str_in]  SampleTime=-1
  Gain1 : Gain  Gain=1/20
  MATLAB Function : MATLAB Function  TreatAsAtomicUnit=on
  MATLAB Function1 : MATLAB Function  TreatAsAtomicUnit=on
  PARSa : Constant  Value=PARSa
  PID Controller : slpidlib/PID Controller  Controller=PID  Form=Parallel  TimeDomain=Discrete-time  UseExternalTs=off  SampleTime=-1  IntegratorMethod=Forward Euler  FilterMethod=Forward Euler  ControllerParametersSource=internal  P=KPspd  I=KIspd  UseKiTs=off  D=KDspd  N=Nspd  UseFilter=on  TunerSelectOption=Transfer Function Based (PID Tuner App)  InitialConditionSource=internal  InitialConditionForIntegrator=0  InitialConditionForFilter=0  DifferentiatorICPrevScaledInput=0  ExternalReset=none  TrackingMode=off  Kt=1  LimitOutput=on  SatLimitsSource=internal  UpperSaturationLimit=Uspd  LowerSaturationLimit=Lspd  LinearizeAsGain=on  AntiWindupMode=clamping  Kb=1  LimitIntegrator=off  UpperIntegratorSaturationLimit=inf  LowerIntegratorSaturationLimit=-inf  POutMin=[]  POutMax=[]  IOutMin=[]  IOutMax=[]  DOutMin=[]  DOutMax=[]  NOutMin=[]  NOutMax=[]  SumOutMin=[]  SumOutMax=[]  SaturationOutMin=[]  SaturationOutMax=[]  PParamMin=[]  PParamMax=[]  IParamMin=[]  IParamMax=[]  DParamMin=[]  DParamMax=[]  NParamMin=[]  NParamMax=[]  KbParamMin=[]  KbParamMax=[]  KtParamMin=[]  KtParamMax=[]  KbOutMin=[]  KbOutMax=[]  KtOutMin=[]  KtOutMax=[]  IntegratorOutMin=[]  IntegratorOutMax=[]  FilterOutMin=[]  FilterOutMax=[]  SumI1OutMin=[]  SumI1OutMax=[]  SumI2OutMin=[]  SumI2OutMax=[]  SumI3OutMin=[]  SumI3OutMax=[]  SumI4OutMin=[]  SumI4OutMax=[]  SumDOutMin=[]  SumDOutMax=[]  DifferentiatorOutMin=[]  DifferentiatorOutMax=[]  FilterDiffOutCoefMin=[]  FilterDiffOutCoefMax=[]  ReciprocalOutMin=[]  ReciprocalOutMax=[]  SumDenOutMin=[]  SumDenOutMax=[]  SumNumOutMin=[]  SumNumOutMax=[]  DivideOutMin=[]  DivideOutMax=[]  UdiffTsProdOutMin=[]  UdiffTsProdOutMax=[]  NTsProdOutMin=[]  NTsProdOutMax=[]  UintegralTsProdOutMin=[]  UintegralTsProdOutMax=[]  UngainTsProdOutMin=[]  UngainTsProdOutMax=[]  ClampingZeroOutDataTypeStr=Inherit: Inherit via back propagation  ClampingZeroOutMin=[]  ClampingZeroOutMax=[]  FilterDenConstantOutDataTypeStr=Inherit: Inherit via back propagation  FilterDenConstantOutMin=[]  FilterDenConstantOutMax=[]  PCopyOutDataTypeStr=Inherit: Inherit via back propagation  PCopyOutMin=[]  PCopyOutMax=[]  NCopyOutDataTypeStr=Inherit: Inherit via back propagation  NCopyOutMin=[]  NCopyOutMax=[]  IntegratorContinuousStateAttributes=''  IntegratorStateMustResolveToSignalObject=off  IntegratorRTWStateStorageClass=Auto  FilterContinuousStateAttributes=''  FilterStateMustResolveToSignalObject=off  FilterRTWStateStorageClass=Auto  ParallelPVariant=InternalParameters  IdealPVariant=Disabled  IVariant=InternalParameters  DVariant=InternalParameters  IntegratorVariant=Discrete  SatVariant=Enabled  AWVariant=DiscClampingParallel  PCopyVariant=Disabled  TRVariant=Disabled  FdbkBlocksVariant=Forward  IdealPFdbkVariant=Disabled  SatFdbkVariant=Disabled  DerivativeFilterVariant=ForwardEulerFilter  NVariant=InternalParameters  NCopyVariant=Disabled  FilterICVariant=InternalICsFilter  IntegratorICVariant=InternalICs  ExternalResetVariant=Disabled  TRSumVariant=Passthrough  SumFdbkVariant=Disabled  SumVariant=Sum_PID  TsampFilterVariant=InternalTs  TsampNgainVariant=Passthrough  TsampIntegralVariant=Passthrough  ExternalSaturationOutDataTypeStr=Inherit: Same as second input
  Rate Limiter1 : RateLimiter  RisingSlewLimit=axle_rate_limit  FallingSlewLimit=-axle_rate_limit  SampleTimeMode=inherited
  Scope : Scope
  Sum : Sum  Inputs=|-+
  To Workspace2 : ToWorkspace  VariableName=U_out_single_littles  SampleTime=-1
  To Workspace3 : ToWorkspace  Commented=on  VariableName=tdig_out_single_littles  SampleTime=-1
  getU : MATLAB Function  TreatAsAtomicUnit=on
  steer : Outport
  Fx_input : Outport  Port=2  VectorParamsAs1DForOutWhenUnconnected=off
  wires:
  q_in/1 -> getU/1(q)
  qd_in/1 -> getU/2(qd)
  getU/1(U) -> To Workspace2/1, Sum/1
  Digital Clock1/1 -> To Workspace3/1
  From Workspace/1 -> Gain1/1
  Gain1/1 -> Scope/1, MATLAB Function/1(str1)
  MATLAB Function/1(y) -> Rate Limiter1/1
  Constant3/1 -> MATLAB Function/2(PARSa)
  Rate Limiter1/1 -> steer/1
  MATLAB Function1/1(y) -> Fx_input/1
  " PARSu"/1 -> MATLAB Function1/2(PARSu)
  PARSa/1 -> MATLAB Function1/3(PARSa)
  Sum/1 -> PID Controller/1
  PID Controller/1 -> MATLAB Function1/1(adem)
  Constant2/1 -> Sum/2

== system manual_steer/truckmaker model/TruckMaker/CM_FIRST ==
  Sync_In : Inport
  BusCreator1 : BusCreator  Inputs=8
  BusCreator2 : BusCreator  Inputs=6
  Demux1 : Demux  Outputs=14
      settings: DisplayOption=none
  Environment : S-Function  FunctionName=TM_Sfun  Parameters='Environment'  SFunctionDeploymentMode=off  EnableBusSupport=off
  IoIn : S-Function  FunctionName=TM_Sfun  Parameters='IoIn'  SFunctionDeploymentMode=off  EnableBusSupport=off
  Terminator : Terminator
  Sync_Out : Outport
  Env.Misc : Outport  Port=2
  wires:
  BusCreator2/1 -> Terminator/1  "IF Environment (in)"
  BusCreator1/1 -> Env.Misc/1
  Demux1/14 -> BusCreator2/6  "Env sRoad"
  Demux1/13 -> BusCreator2/5  "Env PoI_GCS Elev"
  Demux1/12 -> BusCreator2/4  "Env PoI_GCS Lat"
  Demux1/11 -> BusCreator2/3  "Env PoI_GCS Long"
  Demux1/10 -> BusCreator2/2  "Env Time"
  Demux1/9 -> BusCreator2/1  "Env yDay"
  Demux1/8 -> BusCreator1/8  "Env WindVel_tot z"
  Demux1/7 -> BusCreator1/7  "Env WindVel_tot y"
  Demux1/6 -> BusCreator1/6  "Env WindVel_tot x"
  Demux1/5 -> BusCreator1/5  "Env SolarRadiation"
  Demux1/4 -> BusCreator1/4  "Env AirHumidity"
  Demux1/3 -> BusCreator1/3  "Env AirPressure"
  Demux1/2 -> BusCreator1/2  "Env AirDensity"
  Demux1/1 -> BusCreator1/1  "Env Temperature"
  Environment/2 -> Demux1/1
  Environment/1 -> Sync_Out/1
  IoIn/1 -> Environment/1
  Sync_In/1 -> IoIn/1

== system manual_steer/truckmaker model/TruckMaker/CM_LAST ==
  Sync_In : Inport
  CM_User : S-Function  FunctionName=TM_Sfun  Parameters='CM_User'  SFunctionDeploymentMode=off  EnableBusSupport=off
  IoOut : S-Function  FunctionName=TM_Sfun  Parameters='IoOut'  SFunctionDeploymentMode=off  EnableBusSupport=off
  Sync_Out : Outport
  wires:
  IoOut/1 -> Sync_Out/1
  CM_User/1 -> IoOut/1
  Sync_In/1 -> CM_User/1

== system manual_steer/truckmaker model/TruckMaker/DrivMan ==
  note: There's rarely a reason to override DrivMan signals.
      | Use the VehicleControl interface for this purpose.
  Sync_In : Inport
  Env.Misc : Inport  Port=2
  BusCreator : BusCreator  Inputs=17
  Demux : Demux  Outputs=17
      settings: DisplayOption=none
  DrivMan : S-Function  FunctionName=TM_Sfun  Parameters='DrivMan'  SFunctionDeploymentMode=off  EnableBusSupport=off
  Sync_Out : Outport
  DrivMan.Out : Outport  Port=2
  wires:
  Demux/17 -> BusCreator/17  "DrivMan Steering Trq"
  Demux/16 -> BusCreator/16  "DrivMan Steering AngAcc"
  Demux/15 -> BusCreator/15  "DrivMan Steering AngVel"
  Demux/14 -> BusCreator/14  "DrivMan Steering Ang"
  Demux/13 -> BusCreator/13  "DrivMan Gas"
  Demux/12 -> BusCreator/12  "DrivMan Clutch"
  Demux/11 -> BusCreator/11  "DrivMan BrakePark"
  Demux/10 -> BusCreator/10  "DrivMan Brake"
  Demux/9 -> BusCreator/9  "DrivMan GearNo"
  Demux/8 -> BusCreator/8  "DrivMan SelectorCtrl"
  Demux/7 -> BusCreator/7  "DrivMan UserSignal4"
  Demux/6 -> BusCreator/6  "DrivMan UserSignal3"
  Demux/5 -> BusCreator/5  "DrivMan UserSignal2"
  Demux/4 -> BusCreator/4  "DrivMan UserSignal1"
  Demux/3 -> BusCreator/3  "DrivMan UserSignal0"
  Demux/2 -> BusCreator/2  "DrivMan Key"
  Demux/1 -> BusCreator/1  "DrivMan SST"
  Env.Misc/1 -> DrivMan/2
  Sync_In/1 -> DrivMan/1
  DrivMan/1 -> Sync_Out/1
  BusCreator/1 -> DrivMan.Out/1
  DrivMan/2 -> Demux/1

== system manual_steer/truckmaker model/TruckMaker/IPG Vehicle ==
  Sync_In : Inport
  Vhcl.Model.Source : Inport  Port=2
  VhclCtrl.Steering : Inport  Port=3
  Vhcl.Wheel.In : Inport  Port=4
  Vhcl.Misc : Inport  Port=5
  VhclCtrl.Brake : Inport  Port=6
  VhclCtrl.PT : Inport  Port=7
  AFGc : Subsystem
  Brake : Subsystem
  CarAndTrailer : Subsystem
  PowerTrain : Subsystem
  Stop Simulation : Stop
  VehicleSource_BuiltIn : simulink/Logic and Bit Operations/Compare To Constant  relop=~=  const=1  OutDataTypeStr=boolean  ZeroCross=off
  Sync_Out : Outport
  wires:
  VhclCtrl.PT/1 -> PowerTrain/3(VhclCtrl.PT)
  Brake/1(Sync_Out) -> PowerTrain/1(Sync_In)
  CarAndTrailer/1(Sync_Out) -> Brake/1(Sync_In)
  CarAndTrailer/2(Brake.IF.In) -> Brake/2(Brake.IF.In)
  VhclCtrl.Brake/1 -> Brake/3(VhclCtrl.Brake)
  PowerTrain/1(Sync_Out) -> Sync_Out/1
  Vhcl.Misc/1 -> CarAndTrailer/4(Vhcl.Misc)
  Vhcl.Wheel.In/1 -> CarAndTrailer/3(Vhcl.Wheel.In)
  VhclCtrl.Steering/1 -> CarAndTrailer/2(VhclCtrl.Steering)
  Sync_In/1 -> CarAndTrailer/1(Sync_In)
  Vhcl.Model.Source/1 -> VehicleSource_BuiltIn/1
  VehicleSource_BuiltIn/1 -> Stop Simulation/1
  Brake/2(Vhcl.Wheel.PT) -> PowerTrain/2(Vhcl.Wheel.PT)
  AFGc/1(tractor brake) -> Brake/4(tractor brake)
